simulink model "simple_custom_mask"  (Simulink 7.1)
settings: Solver=ode45  StartTime=0.0  StopTime=10.0  RelTol=1e-3
settings Model: Creator=Administrator  LastModifiedBy=Administrator

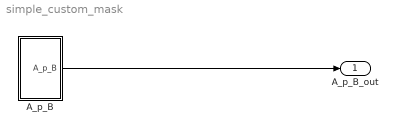
== system simple_custom_mask ==
  A_p_B : Subsystem  mask{A=3, B=10.2}
      mask prompts: A "Enter A:"; B "Enter B:"
  A_p_B_out : Outport  OutDataType=sfix(16)  OutScaling=2^0
  wires:
  A_p_B/1(A_p_B) -> A_p_B_out/1

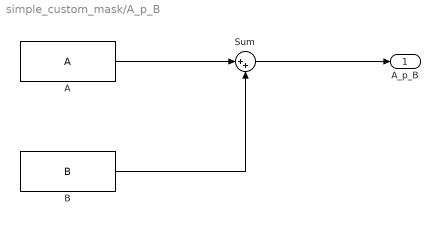
== system simple_custom_mask/A_p_B ==
  A : Constant  Value=A  OutDataType=sfix(16)  OutScaling=2^0
  B : Constant  Value=B  OutDataType=sfix(16)  OutScaling=2^0
  Sum : Sum  Inputs=|++  OutDataType=sfix(16)  OutScaling=2^0
  A_p_B : Outport  OutDataType=sfix(16)  OutScaling=2^0
  wires:
  A/1 -> Sum/1
  B/1 -> Sum/2
  Sum/1 -> A_p_B/1
